simulink subsystem "Stabilisationsregler_side"  (R2023a)
settings: Solver=VariableStepAuto  StartTime=0.0  StopTime=10.0  RelTol=1e-3
undefined symbols (not defined in the file): DiscIntNeverNeededParam, F_int_side, F_side, G_side
settings Model: Creator=morit  LastModifiedBy=morit

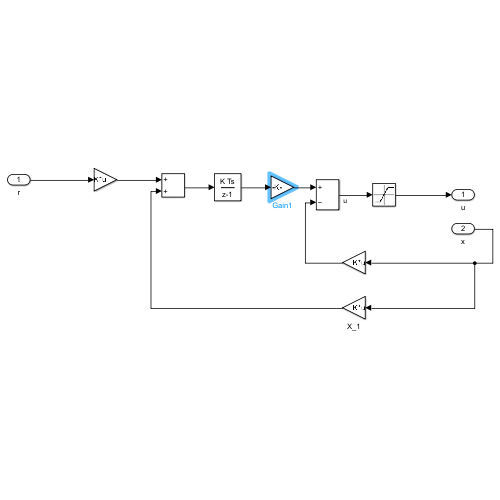
[thumbnail: Simulink's stored preview of the top-level diagram]
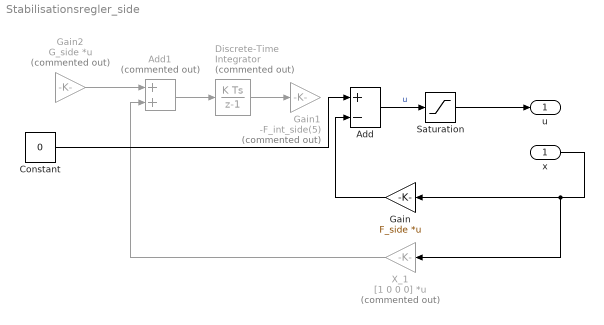
== system Stabilisationsregler_side ==
  x : Inport
  Add : Sum  Inputs=+-
  Add1 : Sum  Commented=on
  Constant : Constant  Value=0
  Discrete-Time Integrator : DiscreteIntegrator  Commented=on  SampleTime=-1  ICPrevOutput=DiscIntNeverNeededParam  ICPrevScaledInput=DiscIntNeverNeededParam
  Gain : Gain  Gain=F_side  Multiplication=Matrix(K*u)
  Gain1 : Gain  Commented=on  Gain=-F_int_side(5)
  Gain2 : Gain  Commented=on  Gain=G_side  Multiplication=Matrix(K*u)
  Saturation : Saturate  UpperLimit=9  LowerLimit=-9
  X_1 : Gain  Commented=on  Gain=[1 0 0 0]  Multiplication=Matrix(K*u)
  u : Outport
  wires:
  Add1/1 -> Discrete-Time Integrator/1
  Discrete-Time Integrator/1 -> Gain1/1
  Gain2/1 -> Add1/1
  X_1/1 -> Add1/2
  Gain/1 -> Add/2
  Add/1 -> Saturation/1  "u"
  x/1 -> Gain/1, X_1/1
  ? -> Gain2/1
  Saturation/1 -> u/1
  Constant/1 -> Add/1
